simulink library "common_lib"  (R2021b)
settings: Solver=ode45  StartTime=0.0  StopTime=10.0  RelTol=1e-3
undefined symbols (not defined in the file or in its folder): ACCEL_PRE_MULT, C_C1GearNumbers, C_C1GearRatios, C_Calibration, C_DitherWaveform, C_GearOffset, C_GearRatioIn, C_GearRatioInverseOut, C_GearRatioOut, CLUTCH_INNER_LOOP_UPDATE_RATE, CONSTANT, DEGRADED_MODE_SIZE, Dem_EventStatusType, DiscIntNeverNeededParam, F_FAULT_ENUM, F_NOFAULT, F_OUTOFRANGE, F_RATELIMIT, FALSE, FMI14_SPECIAL_INSTRUCTIONS, FMI20_DATA_DRIFTED_HIGH, FMI21_DATA_DRIFTED_LOW, FMI29_RESERVED_FOR_SAE_ASSIGNMENT, FMI30_RESERVED_FOR_SAE_ASSIGNMENT, FMI31_CONDITION_EXISTS, FMI32_NO_FAULT, IC, k_accel, k_mean, LVDCU_OORH_FaultCntThd_C, MAX_UINT32, MEAN_PRE_MULT, NTriggers, QLTY_SIGNAL_FAILED, QLTY_SIGNAL_FULLY_FUNCTION, QLTY_SIGNAL_SUBSTITUTED_BY_1ST_CHOICE, QLTY_SIGNAL_SUBSTITUTED_BY_2ND_CHOICE, QLTY_SIGNAL_SUBSTITUTED_BY_3RD_CHOICE, QLTY_SIGNAL_SUBSTITUTED_BY_4TH_CHOICE, SAMPLE_TIME_100_mSec, SAMPLE_TIME_100_uSec, simin, T_TestPoint, TF_FALSE, TF_TRUE, TimeStep, TRUE, WORKSPACE_UPDATE_RATE, ZERO, Zero
libraries: $bdroot x120, simulink x27, simulink_extras x4, MBD_EPS_Local_Blockset x4
(part 4 of 10)

== system common_lib/Ctrl/Dither w Reset ==
  note: Filter output waveform to smooth
      | the transitions if necessary.
  note: Keep present output state until
      | number of executions has occured.
      | (initialize to FALSE)
  note: Keep track of number of iterations
      | since last output transition.
      | (initialize to zero)
  note: Calculate number of executions
      | between alternating output.
      | 1/ (2 * TimeStep * frequency)
      | Add in half a frame to roundoff to
      | nearest minor frame boundary
  note: Simple Dither Function
      | Outputs a modified rectangular wave of specified
      | amplitude, frequency and filter constant.  Also
      | provides a reset signal on switch of output sign.
  note: Common Library::Dither with Reset
  amplitude : Inport
  frequency : Inport  Port=2
  tau : Inport  Port=3
  Constant1 : Constant  Value=MinusOne
  Constant14 : Constant  Value=int16(1)
  Constant2 : Constant  Value=One
  Constant3 : Constant  Value=Two
  Constant4 : Constant  Value=One
  Constant5 : Constant  Value=lim
  Constant6 : Constant  Value=One
  Constant7 : Constant  Value=int16(1)
  Constant8 : Constant  Value=TimeStep
  Constant9 : Constant  Value=ZeroFive
  Data Type Conversion : DataTypeConversion  OutDataTypeStr=single  RndMeth=Zero
  Data Type Conversion1 : DataTypeConversion  OutDataTypeStr=single
  Fltr : $bdroot/Fltrs/Fltr  TimeStep=TimeStep
  Logical Operator : Logic  Operator=NOT
  Logical Operator1 : Logic  Operator=NOT
  MinMax1 : MinMax  Inputs=2  InputSameDT=on  SaturateOnIntegerOverflow=on  ZeroCross=off
  MinMax2 : MinMax  Function=max  Inputs=2  InputSameDT=on  SaturateOnIntegerOverflow=on  ZeroCross=off
  Product1 : Product  Inputs=**  InputSameDT=on  OutDataTypeStr=Inherit: Same as first input
  Product2 : Product  Inputs=***  InputSameDT=on  OutDataTypeStr=Inherit: Same as first input
  Product3 : Product  Inputs=*/  InputSameDT=on  OutDataTypeStr=Inherit: Same as first input
  Relational Operator : RelationalOperator  Operator=<  ZeroCross=off  RndMeth=Nearest  InputSameDT=on
  Sum1 : Sum  Inputs=|++  InputSameDT=on  OutDataTypeStr=Inherit: Same as first input
  Sum3 : Sum  Inputs=++|  InputSameDT=on  OutDataTypeStr=Inherit: Same as first input
  Switch1 : Switch  Threshold=0.5  ZeroCross=off  InputSameDT=on
  Switch2 : Switch  Threshold=0.5  ZeroCross=off  InputSameDT=on
  Switch3 : Switch  Threshold=0.5  ZeroCross=off  InputSameDT=on
  Unit Delay1 : UnitDelay  InitialCondition=int16(0)  SampleTime=-1  HasFrameUpgradeWarning=on
  Unit Delay11 : UnitDelay  InitialCondition=false  SampleTime=-1  HasFrameUpgradeWarning=on
  output : Outport  VectorParamsAs1DForOutWhenUnconnected=off
  reset : Outport  Port=2  VectorParamsAs1DForOutWhenUnconnected=off
  wires:
  Constant8/1 -> Data Type Conversion1/1
  Data Type Conversion1/1 -> Product2/1
  Constant9/1 -> Sum1/2
  Sum1/1 -> Relational Operator/2
  Data Type Conversion/1 -> Relational Operator/1
  Relational Operator/1 -> Logical Operator1/1, Switch1/2, Switch3/2
  Product3/1 -> Sum1/1
  Logical Operator/1 -> Switch1/3
  Sum3/1 -> Data Type Conversion/1, Switch3/1
  Constant7/1 -> Sum3/1
  Unit Delay1/1 -> Sum3/2
  Constant14/1 -> Switch3/3
  Switch3/1 -> Unit Delay1/1
  Constant3/1 -> Product2/3
  Constant6/1 -> Product3/1
  MinMax2/1 -> Product3/2
  Fltr/1 -> output/1
  Constant5/1 -> MinMax2/2
  MinMax1/1 -> MinMax2/1
  Constant4/1 -> MinMax1/2
  Product2/1 -> MinMax1/1
  frequency/1 -> Product2/2
  amplitude/1 -> Product1/1
  Switch2/1 -> Product1/2
  Constant2/1 -> Switch2/1
  Constant1/1 -> Switch2/3
  Product1/1 -> Fltr/1
  Switch1/1 -> Switch2/2, Unit Delay11/1
  Unit Delay11/1 -> Switch1/1, Logical Operator/1
  tau/1 -> Fltr/2
  Logical Operator1/1 -> reset/1

== system common_lib/Ctrl/Integrator ==
  note: Common Library::Integral
  input : Inport
  ulim : Inport  Port=2
  llim : Inport  Port=3
  ic : Inport  Port=4
  reset? : Inport  Port=5  OutDataTypeStr=boolean
  Constant1 : Constant  Value=TimeStep
  Data Type Conversion : DataTypeConversion  OutDataTypeStr=single
  Product1 : Product  Inputs=**  InputSameDT=on  OutDataTypeStr=Inherit: Same as first input
  Sat : $bdroot/Slink/Sat
  Sum : Sum  Inputs=++|  InputSameDT=on  OutDataTypeStr=Inherit: Same as first input
  Switch : Switch  Threshold=0.5  ZeroCross=off  InputSameDT=on
  Unit Delay : UnitDelay  InitialCondition=IC  SampleTime=-1  HasFrameUpgradeWarning=on
  Output : Outport  VectorParamsAs1DForOutWhenUnconnected=off
  wires:
  Constant1/1 -> Data Type Conversion/1
  Data Type Conversion/1 -> Product1/1
  Sat/1 -> Unit Delay/1, Output/1
  Unit Delay/1 -> Sum/1
  Switch/1 -> Sat/1
  Sum/1 -> Switch/3
  llim/1 -> Sat/3
  ulim/1 -> Sat/2
  reset?/1 -> Switch/2
  Product1/1 -> Sum/2
  ic/1 -> Switch/1
  input/1 -> Product1/2

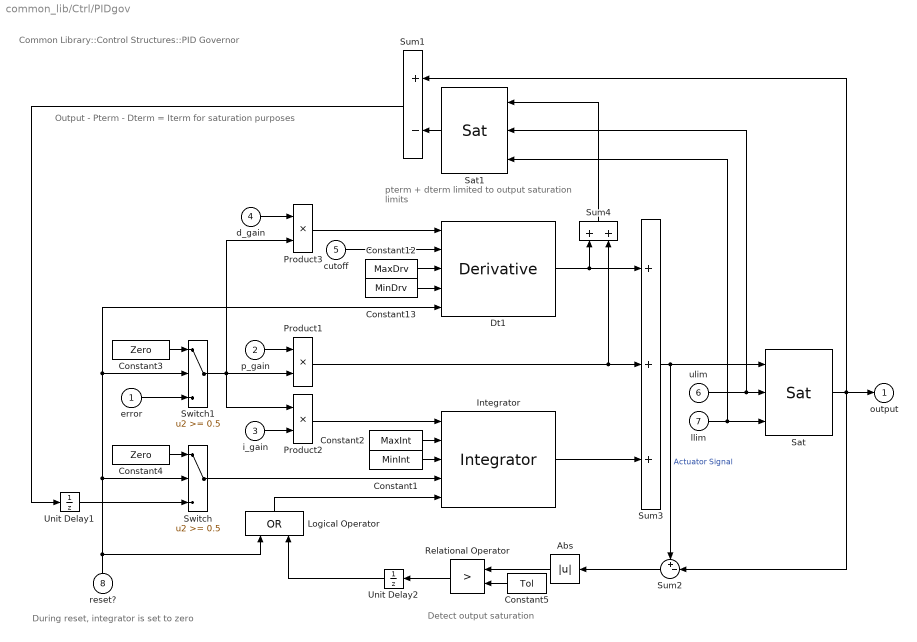
== system common_lib/Ctrl/PIDgov ==
  note: pterm + dterm
      | limited to output saturation limits
  note: Common Library::Control Structures::PID Governor
  note: Detect output saturation
  note: Output - Pterm - Dterm = Iterm for saturation purposes
  note: During reset, integrator is set to zero
  error : Inport
  p_gain : Inport  Port=2
  i_gain : Inport  Port=3
  d_gain : Inport  Port=4
  cutoff : Inport  Port=5
  ulim : Inport  Port=6
  llim : Inport  Port=7
  reset? : Inport  Port=8  OutDataTypeStr=boolean
  Abs : Abs  ZeroCross=off
  Constant1 : Constant  Value=MinInt
  Constant12 : Constant  Value=MaxDrv
  Constant13 : Constant  Value=MinDrv
  Constant2 : Constant  Value=MaxInt
  Constant3 : Constant  Value=Zero
  Constant4 : Constant  Value=Zero
  Constant5 : Constant  Value=Tol
  Dt1 : $bdroot/Ctrl/Derivative  TimeStep=TimeStep
  Integrator : $bdroot/Ctrl/Integrator  TimeStep=TimeStep  IC=IC
  Logical Operator : Logic  Operator=OR
  Product1 : Product  InputSameDT=on  OutDataTypeStr=Inherit: Same as first input
  Product2 : Product  InputSameDT=on  OutDataTypeStr=Inherit: Same as first input
  Product3 : Product  InputSameDT=on  OutDataTypeStr=Inherit: Same as first input
  Relational Operator : RelationalOperator  Operator=>  ZeroCross=off  RndMeth=Nearest  InputSameDT=on
  Sat : $bdroot/Slink/Sat
  Sat1 : $bdroot/Slink/Sat
  Sum1 : Sum  Inputs=+-  InputSameDT=on  OutDataTypeStr=Inherit: Same as first input
  Sum2 : Sum  Inputs=+-|  InputSameDT=on  OutDataTypeStr=Inherit: Same as first input
  Sum3 : Sum  Inputs=+++  InputSameDT=on  OutDataTypeStr=Inherit: Same as first input
  Sum4 : Sum  InputSameDT=on  OutDataTypeStr=Inherit: Same as first input
  Switch : Switch  Threshold=0.5  ZeroCross=off  InputSameDT=on
  Switch1 : Switch  Threshold=0.5  ZeroCross=off  InputSameDT=on
  Unit Delay1 : UnitDelay  InitialCondition=Zero  SampleTime=-1  HasFrameUpgradeWarning=on
      settings: AttributesFormatString=ic=%<X0>
  Unit Delay2 : UnitDelay  InitialCondition=false  SampleTime=-1  HasFrameUpgradeWarning=on
      settings: AttributesFormatString=ic=%<X0>
  output : Outport  InitialOutput=8.973  VectorParamsAs1DForOutWhenUnconnected=off
  wires:
  Switch1/1 -> Product1/2, Product2/1, Product3/2
  error/1 -> Switch1/3
  Constant3/1 -> Switch1/1
  cutoff/1 -> Dt1/2
  Constant12/1 -> Dt1/3
  Constant13/1 -> Dt1/4
  Sat1/1 -> Sum1/2
  Sum4/1 -> Sat1/1
  Dt1/1 -> Sum3/1, Sum4/1
  Unit Delay1/1 -> Switch/3
  Sum2/1 -> Abs/1
  Relational Operator/1 -> Unit Delay2/1
  Abs/1 -> Relational Operator/1
  Constant5/1 -> Relational Operator/2
  Constant2/1 -> Integrator/2
  Constant1/1 -> Integrator/3
  reset?/1 -> Switch1/2, Dt1/5, Switch/2, Logical Operator/1
  ulim/1 -> Sat1/2, Sat/2
  p_gain/1 -> Product1/1
  Product1/1 -> Sum3/2, Sum4/2
  llim/1 -> Sat1/3, Sat/3
  Sum3/1 -> Sat/1, Sum2/1  "Actuator Signal"
  Sat/1 -> Sum1/1, output/1, Sum2/2
  i_gain/1 -> Product2/2
  Constant4/1 -> Switch/1
  Logical Operator/1 -> Integrator/5
  Unit Delay2/1 -> Logical Operator/2
  Switch/1 -> Integrator/4
  Integrator/1 -> Sum3/3
  Sum1/1 -> Unit Delay1/1
  Product2/1 -> Integrator/1
  Product3/1 -> Dt1/1
  d_gain/1 -> Product3/1

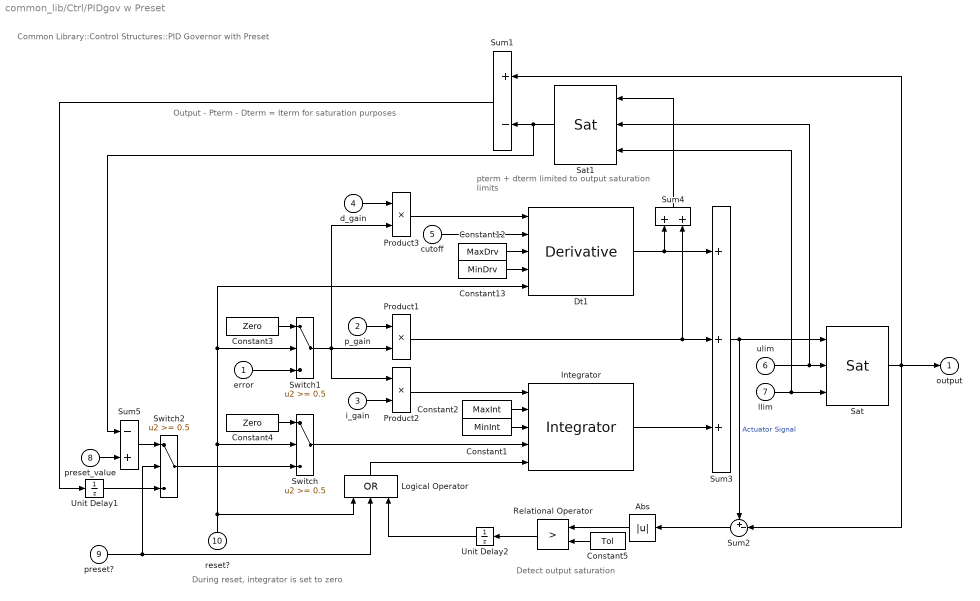
== system common_lib/Ctrl/PIDgov w Preset ==
  note: pterm + dterm
      | limited to output saturation limits
  note: Common Library::Control Structures::PID Governor with Preset
  note: Detect output saturation
  note: Output - Pterm - Dterm = Iterm for saturation purposes
  note: During reset, integrator is set to zero
  error : Inport
  p_gain : Inport  Port=2
  i_gain : Inport  Port=3
  d_gain : Inport  Port=4
  cutoff : Inport  Port=5
  ulim : Inport  Port=6
  llim : Inport  Port=7
  preset_value : Inport  Port=8
  preset? : Inport  Port=9
  reset? : Inport  Port=10  OutDataTypeStr=boolean
  Abs : Abs  ZeroCross=off
  Constant1 : Constant  Value=MinInt
  Constant12 : Constant  Value=MaxDrv
  Constant13 : Constant  Value=MinDrv
  Constant2 : Constant  Value=MaxInt
  Constant3 : Constant  Value=Zero
  Constant4 : Constant  Value=Zero
  Constant5 : Constant  Value=Tol
  Dt1 : $bdroot/Ctrl/Derivative  TimeStep=TimeStep
  Integrator : $bdroot/Ctrl/Integrator  TimeStep=TimeStep  IC=IC
  Logical Operator : Logic  Operator=OR  Inputs=3
  Product1 : Product  InputSameDT=on  OutDataTypeStr=Inherit: Same as first input
  Product2 : Product  InputSameDT=on  OutDataTypeStr=Inherit: Same as first input
  Product3 : Product  InputSameDT=on  OutDataTypeStr=Inherit: Same as first input
  Relational Operator : RelationalOperator  Operator=>  ZeroCross=off  RndMeth=Nearest  InputSameDT=on
  Sat : $bdroot/Slink/Sat
  Sat1 : $bdroot/Slink/Sat
  Sum1 : Sum  Inputs=+-  InputSameDT=on  OutDataTypeStr=Inherit: Same as first input
  Sum2 : Sum  Inputs=+-|  InputSameDT=on  OutDataTypeStr=Inherit: Same as first input
  Sum3 : Sum  Inputs=+++  InputSameDT=on  OutDataTypeStr=Inherit: Same as first input
  Sum4 : Sum  InputSameDT=on  OutDataTypeStr=Inherit: Same as first input
  Sum5 : Sum  Inputs=-+  InputSameDT=on  OutDataTypeStr=Inherit: Same as first input
  Switch : Switch  Threshold=0.5  ZeroCross=off  InputSameDT=on
  Switch1 : Switch  Threshold=0.5  ZeroCross=off  InputSameDT=on
  Switch2 : Switch  Threshold=0.5  ZeroCross=off  InputSameDT=on
  Unit Delay1 : UnitDelay  InitialCondition=Zero  SampleTime=-1  HasFrameUpgradeWarning=on
      settings: AttributesFormatString=ic=%<X0>
  Unit Delay2 : UnitDelay  InitialCondition=false  SampleTime=-1  HasFrameUpgradeWarning=on
      settings: AttributesFormatString=ic=%<X0>
  output : Outport  InitialOutput=8.973  VectorParamsAs1DForOutWhenUnconnected=off
  wires:
  Sum5/1 -> Switch2/1
  preset_value/1 -> Sum5/2
  Switch2/1 -> Switch/3
  Unit Delay1/1 -> Switch2/3
  Switch1/1 -> Product1/2, Product2/1, Product3/2
  error/1 -> Switch1/3
  Constant3/1 -> Switch1/1
  cutoff/1 -> Dt1/2
  Constant12/1 -> Dt1/3
  Constant13/1 -> Dt1/4
  preset?/1 -> Switch2/2, Logical Operator/2
  Sat1/1 -> Sum5/1, Sum1/2
  Sum4/1 -> Sat1/1
  Dt1/1 -> Sum3/1, Sum4/1
  Sum2/1 -> Abs/1
  Relational Operator/1 -> Unit Delay2/1
  Abs/1 -> Relational Operator/1
  Constant5/1 -> Relational Operator/2
  Constant2/1 -> Integrator/2
  Constant1/1 -> Integrator/3
  reset?/1 -> Switch1/2, Dt1/5, Switch/2, Logical Operator/1
  ulim/1 -> Sat1/2, Sat/2
  p_gain/1 -> Product1/1
  Product1/1 -> Sum3/2, Sum4/2
  llim/1 -> Sat1/3, Sat/3
  Sum3/1 -> Sat/1, Sum2/1  "Actuator Signal"
  Sat/1 -> Sum1/1, output/1, Sum2/2
  i_gain/1 -> Product2/2
  Constant4/1 -> Switch/1
  Logical Operator/1 -> Integrator/5
  Unit Delay2/1 -> Logical Operator/3
  Switch/1 -> Integrator/4
  Integrator/1 -> Sum3/3
  Sum1/1 -> Unit Delay1/1
  Product2/1 -> Integrator/1
  Product3/1 -> Dt1/1
  d_gain/1 -> Product3/1

== system common_lib/Ctrl/PIgov ==
  note: pterm
      | limited to output saturation limits
  note: Common Library::Control Structures::PI Governor
  note: Detect output saturation
  note: Output - Pterm - Dterm = Iterm for saturation purposes
  note: During reset, integrator is set to zero
  error : Inport
  p_gain : Inport  Port=2
  i_gain : Inport  Port=3
  ulim : Inport  Port=4
  llim : Inport  Port=5
  reset? : Inport  Port=6  OutDataTypeStr=boolean
  Abs : Abs  ZeroCross=off
  Constant1 : Constant  Value=MinInt
  Constant2 : Constant  Value=MaxInt
  Constant3 : Constant  Value=Zero  OutDataTypeStr=Inherit: Inherit via back propagation
  Constant4 : Constant  Value=Zero  OutDataTypeStr=Inherit: Inherit via back propagation
  Constant5 : Constant  Value=Tol
  Integrator01 : Subsystem  AncestorBlock=common_lib/Ctrl/Integrator  TreatAsAtomicUnit=on  RTWFcnName=INTEGRATOR01  mask(CL Integrator){TimeStep=TimeStep, IC=IC}
      mask prompts: TimeStep "Time Step"; IC "Initial Condition"
      mask help:
      | Determine the integral of the input.
      | If reset is true (1), the integrator is set to the reset condition input.
      |
      | X(1) = input
      | X(2) = upper limit
      | X(3) = lower limit
      | X(4) = reset condition
      | X(5) = reset
      |
      | Y(1) = output
      |
      | Time step is entered via mask parameter.
      | Initial condition is entered via mask parameter.
      |
      | NgEK, Inc.
      settings: RTWFcnNameOpts=User specified  RTWFileNameOpts=Use function name
      mask Help: web(which(['common_lib3.html']))
      mask Display:
      | patch([0.3 0.3 0.7 0.7], [0.35 0.65 0.65 0.35], [255/255 127/255 255/255])
      | disp('Integrator')
      | port_label('input', 1, 'input')
      | port_label('input', 2, 'ulim')
      | port_label('input', 3, 'llim')
      | port_label('input', 4, 'reset_cond')
      | port_label('input', 5, 'reset?')
      | port_label('output', 1, 'output')
  Logical Operator : Logic  Operator=OR
  Product1 : Product  InputSameDT=on  OutDataTypeStr=Inherit: Same as first input
  Product2 : Product  InputSameDT=on  OutDataTypeStr=Inherit: Same as first input
  Relational Operator : RelationalOperator  Operator=>  ZeroCross=off  RndMeth=Nearest  InputSameDT=on
  Sat : $bdroot/Slink/Sat
  Sat1 : $bdroot/Slink/Sat
  Sum1 : Sum  Inputs=+-  InputSameDT=on  OutDataTypeStr=Inherit: Same as first input
  Sum2 : Sum  Inputs=+-|  InputSameDT=on  OutDataTypeStr=Inherit: Same as first input
  Sum3 : Sum  InputSameDT=on  OutDataTypeStr=Inherit: Same as first input
  Switch : Switch  Threshold=0.5  ZeroCross=off  InputSameDT=on
  Switch1 : Switch  Threshold=0.5  ZeroCross=off  InputSameDT=on
  Unit Delay1 : UnitDelay  InitialCondition=Zero  SampleTime=-1  HasFrameUpgradeWarning=on
      settings: AttributesFormatString=ic=%<X0>
  Unit Delay2 : UnitDelay  InitialCondition=false  SampleTime=-1  HasFrameUpgradeWarning=on
      settings: AttributesFormatString=ic=%<X0>
  output : Outport  InitialOutput=8.973  VectorParamsAs1DForOutWhenUnconnected=off
  wires:
  Switch1/1 -> Product1/2, Product2/1
  error/1 -> Switch1/3
  Constant3/1 -> Switch1/1
  Sat1/1 -> Sum1/2
  Unit Delay1/1 -> Switch/3
  Sum2/1 -> Abs/1
  Relational Operator/1 -> Unit Delay2/1
  Abs/1 -> Relational Operator/1
  Constant5/1 -> Relational Operator/2
  Constant2/1 -> Integrator01/2(ulim)
  Constant1/1 -> Integrator01/3(llim)
  reset?/1 -> Logical Operator/1, Switch1/2, Switch/2
  ulim/1 -> Sat1/2, Sat/2
  p_gain/1 -> Product1/1
  Product1/1 -> Sum3/1, Sat1/1
  llim/1 -> Sat1/3, Sat/3
  Sum3/1 -> Sat/1, Sum2/1  "Actuator Signal"
  Sat/1 -> Sum1/1, output/1, Sum2/2
  i_gain/1 -> Product2/2
  Constant4/1 -> Switch/1
  Logical Operator/1 -> Integrator01/5(reset?)
  Unit Delay2/1 -> Logical Operator/2
  Switch/1 -> Integrator01/4(ic)
  Integrator01/1(Output) -> Sum3/2
  Sum1/1 -> Unit Delay1/1
  Product2/1 -> Integrator01/1(input)

== system common_lib/Ctrl/PIgov w Preset ==
  note: pterm
      | limited to output saturation limits
  note: Common Library::Control Structures::PID Governor with Preset
  note: Detect output saturation
  note: Output - Pterm - Dterm = Iterm for saturation purposes
  note: During reset, integrator is set to zero
  error : Inport
  p_gain : Inport  Port=2
  i_gain : Inport  Port=3
  ulim : Inport  Port=4
  llim : Inport  Port=5
  preset_value : Inport  Port=6
  preset? : Inport  Port=7
  reset? : Inport  Port=8  OutDataTypeStr=boolean
  Abs : Abs  ZeroCross=off
  Constant1 : Constant  Value=MinInt
  Constant2 : Constant  Value=MaxInt
  Constant3 : Constant  Value=Zero
  Constant4 : Constant  Value=Zero
  Constant5 : Constant  Value=Tol
  Integrator : $bdroot/Ctrl/Integrator  TimeStep=TimeStep  IC=IC
  Logical Operator : Logic  Operator=OR  Inputs=3
  Product1 : Product  InputSameDT=on  OutDataTypeStr=Inherit: Same as first input
  Product2 : Product  InputSameDT=on  OutDataTypeStr=Inherit: Same as first input
  Relational Operator : RelationalOperator  Operator=>  ZeroCross=off  RndMeth=Nearest  InputSameDT=on
  Sat : $bdroot/Slink/Sat
  Sat1 : $bdroot/Slink/Sat
  Sum1 : Sum  Inputs=+-  InputSameDT=on  OutDataTypeStr=Inherit: Same as first input
  Sum2 : Sum  Inputs=+-|  InputSameDT=on  OutDataTypeStr=Inherit: Same as first input
  Sum3 : Sum  InputSameDT=on  OutDataTypeStr=Inherit: Same as first input
  Sum4 : Sum  Inputs=-+  InputSameDT=on  OutDataTypeStr=Inherit: Same as first input
  Switch : Switch  Threshold=0.5  ZeroCross=off  InputSameDT=on
  Switch1 : Switch  Threshold=0.5  ZeroCross=off  InputSameDT=on
  Switch2 : Switch  Threshold=0.5  ZeroCross=off  InputSameDT=on
  Unit Delay1 : UnitDelay  InitialCondition=Zero  SampleTime=-1  HasFrameUpgradeWarning=on
      settings: AttributesFormatString=ic=%<X0>
  Unit Delay2 : UnitDelay  InitialCondition=false  SampleTime=-1  HasFrameUpgradeWarning=on
      settings: AttributesFormatString=ic=%<X0>
  output : Outport  InitialOutput=8.973  VectorParamsAs1DForOutWhenUnconnected=off
  wires:
  Sum4/1 -> Switch2/1
  Switch2/1 -> Switch/3
  preset_value/1 -> Sum4/2
  Unit Delay1/1 -> Switch2/3
  Switch1/1 -> Product1/2, Product2/1
  error/1 -> Switch1/3
  Constant3/1 -> Switch1/1
  preset?/1 -> Switch2/2, Logical Operator/2
  Sat1/1 -> Sum4/1, Sum1/2
  Sum2/1 -> Abs/1
  Relational Operator/1 -> Unit Delay2/1
  Abs/1 -> Relational Operator/1
  Constant5/1 -> Relational Operator/2
  Constant2/1 -> Integrator/2
  Constant1/1 -> Integrator/3
  reset?/1 -> Switch1/2, Switch/2, Logical Operator/1
  ulim/1 -> Sat1/2, Sat/2
  p_gain/1 -> Product1/1
  Product1/1 -> Sum3/1, Sat1/1
  llim/1 -> Sat1/3, Sat/3
  Sum3/1 -> Sat/1, Sum2/1  "Actuator Signal"
  Sat/1 -> Sum1/1, output/1, Sum2/2
  i_gain/1 -> Product2/2
  Constant4/1 -> Switch/1
  Logical Operator/1 -> Integrator/5
  Unit Delay2/1 -> Logical Operator/3
  Switch/1 -> Integrator/4
  Integrator/1 -> Sum3/2
  Sum1/1 -> Unit Delay1/1
  Product2/1 -> Integrator/1

== system common_lib/Ctrl/Ramp ==
  note: Common Library::Ramp
  A : Inport
  B : Inport  Port=2
  C : Inport  Port=3
  reset : Inport  Port=4  OutDataTypeStr=boolean
  Constant1 : Constant  Value=TimeStep
  Data Type Conversion : DataTypeConversion  OutDataTypeStr=single
  MinMax1 : MinMax  Function=max  Inputs=2  InputSameDT=on  SaturateOnIntegerOverflow=on  ZeroCross=off
  MinMax2 : MinMax  Function=max  Inputs=2  InputSameDT=on  SaturateOnIntegerOverflow=on  ZeroCross=off
  MinMax3 : MinMax  Inputs=2  InputSameDT=on  SaturateOnIntegerOverflow=on  ZeroCross=off
  Product1 : Product  Inputs=/**  InputSameDT=on  OutDataTypeStr=Inherit: Same as first input
  Sat : $bdroot/Slink/Sat
  Sum : Sum  Inputs=++|  InputSameDT=on  OutDataTypeStr=Inherit: Same as first input
  Sum1 : Sum  Inputs=-|+  InputSameDT=on  OutDataTypeStr=Inherit: Same as first input
  Switch : Switch  Threshold=0.5  ZeroCross=off  InputSameDT=on
  Switch1 : Switch  Threshold=0.5  ZeroCross=off  InputSameDT=on
  Unit Delay : UnitDelay  InitialCondition=Zero  SampleTime=-1  HasFrameUpgradeWarning=on
      settings: AttributesFormatString=ic=%<X0>
  Unit Delay1 : UnitDelay  InitialCondition=Zero  SampleTime=-1  HasFrameUpgradeWarning=on
      settings: AttributesFormatString=ic=%<X0>
  Unit Delay2 : UnitDelay  InitialCondition=true  SampleTime=-1  HasFrameUpgradeWarning=on
      settings: AttributesFormatString=ic=%<X0>
  Output : Outport  VectorParamsAs1DForOutWhenUnconnected=off
  wires:
  Data Type Conversion/1 -> MinMax1/2, Product1/2
  Constant1/1 -> Data Type Conversion/1
  Unit Delay2/1 -> Switch1/2
  reset/1 -> Unit Delay2/1, Switch/2
  Product1/1 -> Sum/2
  Switch1/1 -> Product1/3, Unit Delay1/1
  Sum1/1 -> Switch1/1
  Unit Delay1/1 -> Switch1/3
  MinMax3/1 -> Sat/3
  MinMax2/1 -> Sat/2
  MinMax1/1 -> Product1/1
  C/1 -> MinMax1/1
  Sat/1 -> Unit Delay/1, Output/1
  Unit Delay/1 -> Sum/1
  Switch/1 -> Sat/1
  Sum/1 -> Switch/3
  B/1 -> MinMax2/2, MinMax3/2, Sum1/2
  A/1 -> MinMax3/1, MinMax2/1, Sum1/1, Switch/1

== system common_lib/Ctrl/Subsystem ==
  ClearCntrRqst : Inport
  Increment_Cntr : Inport  Port=2
  HWpd_Input : Inport  Port=3
  Constant15 : Constant  Value=uint32(1)
  Constant16 : Constant  Value=FALSE
  Constant17 : Constant  Value=MAX_UINT32
  Constant18 : Constant  Value=uint32(0)
  Constant19 : Constant  Value=uint32(0)
  Logical Operator9 : Logic  AllPortsSameDT=off
  Relational Operator6 : RelationalOperator  Operator=<  ZeroCross=off  RndMeth=Nearest  InputSameDT=on
  Sum4 : Sum  Inputs=|++  InputSameDT=on  OutDataTypeStr=Inherit: Same as first input
  Switch10 : Switch  Threshold=0.5  ZeroCross=off  InputSameDT=on
  Switch11 : Switch  Threshold=0.5  ZeroCross=off  InputSameDT=on
  Switch12 : Switch  Threshold=0.5  ZeroCross=off  InputSameDT=on
  Unit Delay8 : UnitDelay  InitialCondition=uint32(0)  SampleTime=-1  HasFrameUpgradeWarning=on
      settings: AttributesFormatString=ic=%<X0>
  Unit Delay9 : UnitDelay  InitialCondition=TRUE  SampleTime=-1  HasFrameUpgradeWarning=on
      settings: AttributesFormatString=ic=%<X0>
  CntrUpdate : Outport  VectorParamsAs1DForOutWhenUnconnected=off
  wires:
  Unit Delay8/1 -> Relational Operator6/1, Sum4/2
  Constant17/1 -> Relational Operator6/2
  Constant19/1 -> Switch12/1
  Switch10/1 -> Switch12/3
  Constant18/1 -> Switch11/3
  Constant15/1 -> Switch11/1
  Switch11/1 -> Sum4/1
  Sum4/1 -> Switch10/3
  Unit Delay9/1 -> Switch10/2
  Constant16/1 -> Unit Delay9/1
  Switch12/1 -> Unit Delay8/1, CntrUpdate/1
  Logical Operator9/1 -> Switch11/2
  Increment_Cntr/1 -> Logical Operator9/1
  Relational Operator6/1 -> Logical Operator9/2
  HWpd_Input/1 -> Switch10/1
  ClearCntrRqst/1 -> Switch12/2

== system common_lib/Ctrl/Trajectory ==
  note: Rate increment happens
      | even during reset
  note: Output - Final
  note: Start - Final
  note: Ignore the start_value
      | if it is moving away
      | from the final_value
  note: Reset if the previous value is further
      |                       away than the current start value
      | or if the final limit is smaller than the start limit
      | or if start is active
  note: Pick rate based on distance
      | from final
  note: Pick rate based on distance
      | from original start
  note: Start-CurrentStart
  note: Common Library::Control Structures::Trajectory Control
  start_value : Inport
  final_value : Inport  Port=2
  start_weight : Inport  Port=3
  stop_weight : Inport  Port=4
  start : Inport  Port=5
  Abs{,1,3..5} (5 alike) : Abs  ZeroCross=off
  Constant1 : Constant  Value=MinusOne
  CurrentStart : Subsystem  TreatAsAtomicUnit=on
      settings: RTWSystemCode=Inline
  FinalRLim : Lookup  InputValues=FinalRLimIn  Table=FinalRLimOut  LookUpMeth=Interpolation-Use End Values
  Logical Operator : Logic  Operator=OR  Inputs=3
  Logical Operator1 : Logic  Operator=OR
  MinMax3 : MinMax  Inputs=2  InputSameDT=on  SaturateOnIntegerOverflow=on  ZeroCross=off
  Relational Operator : RelationalOperator  Operator=<  ZeroCross=off  RndMeth=Nearest  InputSameDT=on
  Relational Operator1 : RelationalOperator  Operator=>  ZeroCross=off  RndMeth=Nearest  InputSameDT=on
  Relational Operator2 : RelationalOperator  ZeroCross=off  RndMeth=Nearest  InputSameDT=on
  Start : Subsystem  TreatAsAtomicUnit=on
      settings: RTWSystemCode=Inline
  StartRLim : Lookup  InputValues=StartRLimIn  Table=StartRLimOut  LookUpMeth=Interpolation-Use End Values
  Sum1 : Sum  Inputs=-+  InputSameDT=on  OutDataTypeStr=Inherit: Same as first input
  Sum2 : Sum  Inputs=-+  InputSameDT=on  OutDataTypeStr=Inherit: Same as first input
  Sum3 : Sum  Inputs=+-  InputSameDT=on  OutDataTypeStr=Inherit: Same as first input
  Sum4 : Sum  Inputs=+-  InputSameDT=on  OutDataTypeStr=Inherit: Same as first input
  Sum6 : Sum  Inputs=+-  InputSameDT=on  OutDataTypeStr=Inherit: Same as first input
  Unit Delay1 : UnitDelay  InitialCondition=Zero  SampleTime=-1  HasFrameUpgradeWarning=on
      settings: AttributesFormatString=ic=%<X0>
  Unit Delay2 : UnitDelay  InitialCondition=Zero  SampleTime=-1  HasFrameUpgradeWarning=on
      settings: AttributesFormatString=ic=%<X0>
  Variable Rate Limiter w IC in feedback loop : Subsystem  mask(CL Variable Rate Limiter with Initial Condition){TimeStep=TimeStep, ic=Zero}
      mask prompts: TimeStep "Time Step"; ic "Initial Condition"
      mask help:
      | Variable rate limiter block with Initial Condiiton
      |
      | X(1) = input
      | X(2) = rise rate
      | X(3) = fall rate
      | X(4) = initial condition
      | X(5) = reset?
      |
      | Y(1) = output
      | NgEK, Inc.
      mask Help: web(which(['common_lib38.html']))
      mask Display:
      | patch([0.3 0.3 0.7 0.7], [0.35 0.65 0.65 0.35], [255/255 127/255 255/255])
      | 
      | plot([0 1],[0.5 0.5],[0.5 0.5],[0 1],[0 1],[0 1],[0.7 0.8 0.8],[0.8 0.8 0.7], [0.2 0.2 0.3],[0.3 0.2 0.2])
  transient_split3 : Product  InputSameDT=on  OutDataTypeStr=Inherit: Same as first input
  transient_split5 : Product  InputSameDT=on  OutDataTypeStr=Inherit: Same as first input
  transient_split6 : Product  InputSameDT=on  OutDataTypeStr=Inherit: Same as first input
  output : Outport  VectorParamsAs1DForOutWhenUnconnected=off
  wires:
  Abs5/1 -> Relational Operator2/1
  Sum4/1 -> Abs5/1
  Unit Delay2/1 -> Sum4/1
  Abs4/1 -> Relational Operator2/2
  Sum3/1 -> Abs4/1
  Relational Operator2/1 -> Logical Operator1/1
  Logical Operator1/1 -> CurrentStart/Enable
  CurrentStart/1(out) -> Start/1(in), Sum1/1, Unit Delay2/1, Variable Rate Limiter w IC in feedback loop/4(ic), Sum2/2
  Variable Rate Limiter w IC in feedback loop/1(output) -> Unit Delay1/1, output/1
  Relational Operator1/1 -> Logical Operator/1
  Abs3/1 -> Relational Operator1/1
  Sum6/1 -> Abs3/1
  Logical Operator/1 -> Variable Rate Limiter w IC in feedback loop/5(reset?)
  Unit Delay1/1 -> Sum6/1
  Relational Operator/1 -> Logical Operator/2
  transient_split5/1 -> Variable Rate Limiter w IC in feedback loop/3(fall rate)
  MinMax3/1 -> Variable Rate Limiter w IC in feedback loop/2(rise rate), transient_split5/1
  final_value/1 -> Sum4/2, Sum3/1, Variable Rate Limiter w IC in feedback loop/1(input), Sum6/2, Sum2/1
  transient_split6/1 -> Relational Operator/1, MinMax3/1
  FinalRLim/1 -> transient_split6/2
  Abs1/1 -> Relational Operator1/2, FinalRLim/1
  Sum2/1 -> Abs1/1
  Constant1/1 -> transient_split5/2
  stop_weight/1 -> transient_split6/1
  transient_split3/1 -> Relational Operator/2, MinMax3/2
  StartRLim/1 -> transient_split3/2
  Abs/1 -> StartRLim/1
  Sum1/1 -> Abs/1
  Start/1(out) -> Sum1/2
  start_weight/1 -> transient_split3/1
  start/1 -> Start/Enable, Logical Operator/3, Logical Operator1/2
  start_value/1 -> CurrentStart/1(in), Sum3/2

== system common_lib/Ctrl/VoltageControllerPI ==
  Err : Inport  OutDataTypeStr=single
  reset : Inport  Port=2  OutDataTypeStr=boolean
  b0 : Inport  Port=3  OutDataTypeStr=single
  b1 : Inport  Port=4  OutDataTypeStr=single
  Add : Sum  Inputs=+++  SaturateOnIntegerOverflow=on
  Constant : Constant  Value=0  OutDataTypeStr=single  SampleTime=-1
  Constant1 : Constant  Value=0  OutDataTypeStr=single  SampleTime=-1
  Divide : Product
  Divide1 : Product
  Saturation : Saturate  UpperLimit=ul  LowerLimit=ll  OutDataTypeStr=single
  Switch : Switch  Criteria=u2 > Threshold  Threshold=0.5
  Switch1 : Switch  Criteria=u2 > Threshold  Threshold=0.5
  Unit Delay : UnitDelay  SampleTime=-1  HasFrameUpgradeWarning=on
      settings: AttributesFormatString=ic=%<X0>
  Unit Delay1 : UnitDelay  SampleTime=-1  HasFrameUpgradeWarning=on
      settings: AttributesFormatString=ic=%<X0>
  out : Outport  VectorParamsAs1DForOutWhenUnconnected=off
  wires:
  Unit Delay/1 -> Divide1/1
  Divide/1 -> Add/1
  Divide1/1 -> Add/2
  Add/1 -> Saturation/1
  Saturation/1 -> Unit Delay1/1, out/1
  Unit Delay1/1 -> Switch/3
  Switch/1 -> Add/3
  reset/1 -> [Reset]
  Constant/1 -> Switch/1
  [Reset] -> Switch/2
  Err/1 -> Switch1/3
  Switch1/1 -> Unit Delay/1, Divide/2
  [Reset] -> Switch1/2
  Constant1/1 -> Switch1/1
  b0/1 -> Divide/1
  b1/1 -> Divide1/2

== system common_lib/Diag/CL MinMax Capture ==
  input : Inport
  hold? : Inport  Port=2
  reset? : Inport  Port=3
  Constant : Constant  Value=InitValue  SampleTime=-1
  Logical Operator : Logic  AllPortsSameDT=off
  Logical Operator1 : Logic  Operator=NOT  AllPortsSameDT=off
  Relational Operator : RelationalOperator  Operator=<  ZeroCross=off  RndMeth=Nearest
  Switch : Switch  Threshold=0.5  ZeroCross=off
  Switch1 : Switch  Threshold=0.5  ZeroCross=off
  Unit Delay : UnitDelay  InitialCondition=InitValue  SampleTime=-1  HasFrameUpgradeWarning=on
      settings: AttributesFormatString=ic=%<X0>
  Output Value : Outport  VectorParamsAs1DForOutWhenUnconnected=off
  wires:
  Constant/1 -> Switch/1
  reset?/1 -> Switch/2
  Switch1/1 -> Switch/3
  input/1 -> Switch1/1, Relational Operator/1  "Input"
  Relational Operator/1 -> Logical Operator/2  "Input past previous value"
  hold?/1 -> Logical Operator1/1  "Hold value"
  Logical Operator1/1 -> Logical Operator/1
  Logical Operator/1 -> Switch1/2  "New value"
  Switch/1 -> Unit Delay/1, Output Value/1
  Unit Delay/1 -> Switch1/3, Relational Operator/2  "Previous value"

== system common_lib/Diag/Command Feedback Test ==
  note: Common Library::Diagnostics::Command Feedback Test
  cmd : Inport
  fbk : Inport  Port=2
  tau : Inport  Port=3
  tau_lim : Inport  Port=4
  tau_time : Inport  Port=5
  error_lim : Inport  Port=6
  error_time : Inport  Port=7
  Enable : EnablePort  ZeroCross=off
  CommandFeedbackFaultLogicCore : Subsystem  TreatAsAtomicUnit=on  RTWFcnName=CFT
      settings: RTWFcnNameOpts=User specified  RTWFileNameOpts=Use function name
  Data Type Conversion{1..7} (7 alike) : DataTypeConversion  OutDataTypeStr=single
  Signal Conversion : SignalConversion  ConversionOutput=Contiguous copy  OverrideOpt=on
  Min Value : Outport  VectorParamsAs1DForOutWhenUnconnected=off
  wires:
  cmd/1 -> Data Type Conversion7/1
  tau/1 -> Data Type Conversion5/1
  tau_lim/1 -> Data Type Conversion4/1
  tau_time/1 -> Data Type Conversion3/1
  error_lim/1 -> Data Type Conversion2/1
  CommandFeedbackFaultLogicCore/1(Min Value) -> Signal Conversion/1
  fbk/1 -> Data Type Conversion6/1
  error_time/1 -> Data Type Conversion1/1
  Signal Conversion/1 -> Min Value/1
  Data Type Conversion1/1 -> CommandFeedbackFaultLogicCore/7(error_time)
  Data Type Conversion2/1 -> CommandFeedbackFaultLogicCore/6(error_lim)
  Data Type Conversion3/1 -> CommandFeedbackFaultLogicCore/5(tau_time)
  Data Type Conversion4/1 -> CommandFeedbackFaultLogicCore/4(tau_lim)
  Data Type Conversion5/1 -> CommandFeedbackFaultLogicCore/3(tau)
  Data Type Conversion6/1 -> CommandFeedbackFaultLogicCore/2(fbk)
  Data Type Conversion7/1 -> CommandFeedbackFaultLogicCore/1(cmd)

== system common_lib/Diag/Fault Counter ==
  note: Common Library::Diagnostics::Fault Counter
  fl : Inport  OutDataTypeStr=boolean
  true_count : Inport  Port=2
  false_count : Inport  Port=3
  fc_level : Inport  Port=4
  reset : Inport  Port=5  OutDataTypeStr=boolean
  Compare To Zero : simulink/Logic and Bit Operations/Compare To Zero  relop=>  OutDataTypeStr=boolean  ZeroCross=off
  Constant : Constant  Value=true
  DTC : DataTypeConversion  OutDataTypeStr=boolean
  DTC1 : DataTypeConversion  OutDataTypeStr=boolean
  DTC3 : DataTypeConversion  OutDataTypeStr=int16
  FaultCounter : Subsystem  RTWFcnName=FLTCNTR
      settings: RTWSystemCode=Inline  RTWFcnNameOpts=User specified  RTWFileNameOpts=Use function name
  Logical Operator : Logic  AllPortsSameDT=off  OutDataTypeStr=boolean
  Logical Operator1 : Logic  Operator=OR  AllPortsSameDT=off  OutDataTypeStr=boolean
  Signal Conversion : SignalConversion  ConversionOutput=Contiguous copy  OverrideOpt=on
  Unit Delay : UnitDelay  InitialCondition=ZERO  SampleTime=-1  HasFrameUpgradeWarning=on
      settings: AttributesFormatString=ic=%<X0>
  Unit Delay1 : UnitDelay  InitialCondition=false  SampleTime=-1  HasFrameUpgradeWarning=on
      settings: AttributesFormatString=ic=%<X0>
  inc switch : Switch  Criteria=u2 ~= 0  Threshold=0.5  ZeroCross=off  InputSameDT=on
  fc : Outport  VectorParamsAs1DForOutWhenUnconnected=off
  wires:
  FaultCounter/1(count) -> Unit Delay/1
  Unit Delay/1 -> FaultCounter/2(count_prev), Compare To Zero/1
  fc_level/1 -> DTC3/1
  reset/1 -> DTC1/1
  fl/1 -> DTC/1
  FaultCounter/2(fc) -> Signal Conversion/1
  Logical Operator/1 -> FaultCounter/Enable
  Constant/1 -> Unit Delay1/1
  Unit Delay1/1 -> Logical Operator/2
  Compare To Zero/1 -> Logical Operator1/1
  Logical Operator1/1 -> Logical Operator/1
  Signal Conversion/1 -> fc/1
  DTC/1 -> Logical Operator1/2, inc switch/2
  DTC1/1 -> FaultCounter/4(reset)
  DTC3/1 -> FaultCounter/3(fc_level)
  false_count/1 -> inc switch/3
  true_count/1 -> inc switch/1
  inc switch/1 -> FaultCounter/1(fl)

== system common_lib/Diag/Fault Counter w Hold ==
  note: Common Library::Diagnostics::Fault Counter with Hold
  fl : Inport  OutDataTypeStr=boolean
  hold : Inport  Port=2
  true_count : Inport  Port=3
  false_count : Inport  Port=4
  fc_level : Inport  Port=5
  reset : Inport  Port=6  OutDataTypeStr=boolean
  Constant1 : Constant  Value=ZERO
  Constant2 : Constant  Value=false
  Constant3 : Constant  Value=true
  Constant4 : Constant  Value=ZERO
  Constant5 : Constant  Value=false
  Constant6 : Constant  Value=ZERO
  Logical Operator : Logic  Operator=OR
  Relay : $bdroot/Slink/Relay  init=false
      settings: AttributesFormatString=ic=%<init>
  Sat : $bdroot/Slink/Sat
  Sum : Sum  Inputs=++|  InputSameDT=on  OutDataTypeStr=Inherit: Same as first input
  Unit Delay : UnitDelay  InitialCondition=ZERO  SampleTime=-1  HasFrameUpgradeWarning=on
      settings: AttributesFormatString=ic=%<X0>
  Unit Delay1 : UnitDelay  InitialCondition=true  SampleTime=-1  HasFrameUpgradeWarning=on
      settings: AttributesFormatString=ic=%<X0>
  inc switch : Switch  Threshold=0.5  ZeroCross=off  InputSameDT=on
  inc switch1 : Switch  Threshold=0.5  ZeroCross=off  InputSameDT=on
  reset switch1 : Switch  Threshold=0.5  ZeroCross=off  InputSameDT=on
  fc : Outport  VectorParamsAs1DForOutWhenUnconnected=off
  wires:
  inc switch1/1 -> Sum/2
  Constant4/1 -> inc switch1/1
  hold/1 -> inc switch1/2
  Sum/1 -> reset switch1/3
  Constant6/1 -> reset switch1/1
  Relay/1 -> fc/1
  Constant3/1 -> Relay/4
  Constant2/1 -> Relay/5
  Constant1/1 -> Relay/3, Sat/3
  fc_level/1 -> Relay/2, Sat/2
  Sat/1 -> Unit Delay/1
  inc switch/1 -> inc switch1/3
  true_count/1 -> inc switch/1
  fl/1 -> inc switch/2
  false_count/1 -> inc switch/3
  Constant5/1 -> Unit Delay1/1
  Unit Delay1/1 -> Logical Operator/2
  reset/1 -> Logical Operator/1
  Logical Operator/1 -> reset switch1/2
  Unit Delay/1 -> Sum/1
  reset switch1/1 -> Relay/1, Sat/1

== system common_lib/Diag/Fault Injection ==
  note: Common Library::Diagnostics::Fault Injection
  input : Inport
  gain : Inport  Port=2
  offset : Inport  Port=3
  ulim : Inport  Port=4
  llim : Inport  Port=5
  hold : Inport  Port=6
  fl_trigger : Inport  Port=7
  Gain and Offset (in) : $bdroot/SCond/Gain and Offset (in)  DataType=Double
  OOR Fault Detection : $bdroot/Diag/OOR Fault Detection  InitialValue=InitialValue
  Switch : Switch  Threshold=0.5  ZeroCross=off
  Unit Delay : UnitDelay  InitialCondition=InitialValue  SampleTime=-1  HasFrameUpgradeWarning=on
  output : Outport  VectorParamsAs1DForOutWhenUnconnected=off
  hwfl : Outport  Port=2  VectorParamsAs1DForOutWhenUnconnected=off
  wires:
  Gain and Offset (in)/1 -> Switch/3
  Switch/1 -> OOR Fault Detection/1
  Unit Delay/1 -> Switch/1
  hold/1 -> Switch/2
  llim/1 -> OOR Fault Detection/3
  ulim/1 -> OOR Fault Detection/2
  fl_trigger/1 -> OOR Fault Detection/4
  OOR Fault Detection/2 -> hwfl/1
  OOR Fault Detection/1 -> Unit Delay/1, output/1
  offset/1 -> Gain and Offset (in)/3
  gain/1 -> Gain and Offset (in)/2
  input/1 -> Gain and Offset (in)/1

== system common_lib/Diag/Fault Log ==
  note: Common Library::Diagnostics::Fault Log
  HWfl_Active : Inport  OutDataTypeStr=boolean
  HWfl_Events : Inport  Port=2  OutDataTypeStr=uint16
  HWfl_Frames : Inport  Port=3  OutDataTypeStr=uint32
  hold : Inport  Port=4  OutDataTypeStr=boolean
  Constant1 : Constant  Value=EVENT_ZERO
  Constant18 : Constant  Value=EVENT_MAX
  Constant2 : Constant  Value=EVENT_ONE
  Constant3 : Constant  Value=FRAME_ZERO
  Constant4 : Constant  Value=FRAME_MAX
  Constant5 : Constant  Value=FRAME_ONE
  Logical Operator1 : Logic
  Logical Operator3 : Logic
  Logical Operator8 : Logic
  Sat : $bdroot/Slink/Sat
  Sat1 : $bdroot/Slink/Sat
  Sum : Sum  Inputs=|++  InputSameDT=on  OutDataTypeStr=Inherit: Same as first input
  Sum1 : Sum  Inputs=|++  InputSameDT=on  OutDataTypeStr=Inherit: Same as first input
  Unit Delay1 : UnitDelay  InitialCondition=false  SampleTime=-1  HasFrameUpgradeWarning=on
  not1 : Logic  Operator=NOT
  not2 : Logic  Operator=NOT
  reset switch : Switch  Criteria=u2 ~= 0  Threshold=0.5  ZeroCross=off  InputSameDT=on
  reset switch1 : Switch  Criteria=u2 ~= 0  Threshold=0.5  ZeroCross=off  InputSameDT=on
  events : Outport  VectorParamsAs1DForOutWhenUnconnected=off
  frames : Outport  Port=2  VectorParamsAs1DForOutWhenUnconnected=off
  wires:
  Logical Operator3/1 -> reset switch/2
  Logical Operator8/1 -> not1/1, Logical Operator3/1
  Unit Delay1/1 -> Logical Operator3/2
  not1/1 -> Unit Delay1/1
  Logical Operator1/1 -> reset switch1/2
  hold/1 -> not2/1
  not2/1 -> Logical Operator8/2, Logical Operator1/1
  HWfl_Frames/1 -> Sum1/2, reset switch1/3
  HWfl_Events/1 -> Sum/2, reset switch/3
  Constant5/1 -> Sum1/1
  Sat1/1 -> frames/1
  Sum1/1 -> reset switch1/1
  reset switch1/1 -> Sat1/1
  Constant3/1 -> Sat1/3
  Constant4/1 -> Sat1/2
  Constant2/1 -> Sum/1
  Sat/1 -> events/1
  Sum/1 -> reset switch/1
  reset switch/1 -> Sat/1
  Constant1/1 -> Sat/3
  Constant18/1 -> Sat/2
  HWfl_Active/1 -> Logical Operator1/2, Logical Operator8/1

== system common_lib/Diag/Fault_Cntr ==
  note: Common Library::Diagnostics::Fault Counter
  fl : Inport  OutDataTypeStr=boolean
  reset : Inport  Port=2  OutDataTypeStr=boolean
  fmi : Inport  Port=3  OutDataTypeStr=uint16
  Constant1 : Constant  Value=up_cnt
  Constant10 : Constant  Value=red_light  OutDataTypeStr=boolean
  Constant2 : Constant  Value=dn_cnt
  Constant3 : Constant  Value=fc_level  OutDataTypeStr=int16
  Constant4 : Constant  Value=fault_id  OutDataTypeStr=uint16
  Constant6 : Constant  Value=amber_light  OutDataTypeStr=boolean
  Data Type Conversion : DataTypeConversion  OutDataTypeStr=uint16
  Data Type Conversion1 : DataTypeConversion  OutDataTypeStr=boolean
  Data Type Conversion2 : DataTypeConversion  OutDataTypeStr=int16
  Data Type Conversion3 : DataTypeConversion  OutDataTypeStr=int16
  FaultHandlerCoreLogic : Subsystem  TreatAsAtomicUnit=on  RTWFcnName=FC_FMI_Handler
      settings: RTWFcnNameOpts=User specified  RTWFileNameOpts=Use function name
  Signal Conversion : SignalConversion  ConversionOutput=Contiguous copy  OverrideOpt=on
  Signal Conversion1 : SignalConversion  ConversionOutput=Contiguous copy  OverrideOpt=on
  inc switch : Switch  Criteria=u2 ~= 0  Threshold=0.5  ZeroCross=off  InputSameDT=on
  fc : Outport  OutDataTypeStr=uint16  VectorParamsAs1DForOutWhenUnconnected=off
  lights : Outport  Port=2  OutDataTypeStr=uint8  VectorParamsAs1DForOutWhenUnconnected=off
  wires:
  fl/1 -> inc switch/2
  reset/1 -> Data Type Conversion1/1
  FaultHandlerCoreLogic/1(fc) -> Signal Conversion/1
  fmi/1 -> Data Type Conversion/1
  FaultHandlerCoreLogic/2(lights) -> Signal Conversion1/1
  Signal Conversion/1 -> fc/1
  Signal Conversion1/1 -> lights/1
  Data Type Conversion/1 -> FaultHandlerCoreLogic/3(fmi)
  Data Type Conversion1/1 -> FaultHandlerCoreLogic/2(reset)
  Constant2/1 -> inc switch/3
  Constant3/1 -> Data Type Conversion3/1
  Constant4/1 -> FaultHandlerCoreLogic/5(fid)
  Constant10/1 -> FaultHandlerCoreLogic/6(red)
  Constant6/1 -> FaultHandlerCoreLogic/7(amber)
  Constant1/1 -> inc switch/1
  inc switch/1 -> Data Type Conversion2/1
  Data Type Conversion2/1 -> FaultHandlerCoreLogic/1(fl)
  Data Type Conversion3/1 -> FaultHandlerCoreLogic/4(fc_level)

== system common_lib/Diag/Filter w Fault Handler ==
  input : Inport
  tau : Inport  Port=2
  override_value : Inport  Port=3
  override? : Inport  Port=4
  reset? : Inport  Port=5
  default : Inport  Port=6
  ramp_time : Inport  Port=7
  fault? : Inport  Port=8
  Data Type Conversion{,1..4} (5 alike) : DataTypeConversion  OutDataTypeStr=single
  Data Type Conversion5 : DataTypeConversion  OutDataTypeStr=boolean
  Data Type Conversion6 : DataTypeConversion  OutDataTypeStr=boolean
  Data Type Conversion7 : DataTypeConversion  OutDataTypeStr=boolean
  FilterWithFaultHandlerCoreLogic : Subsystem  TreatAsAtomicUnit=on  RTWFcnName=FLTRWROFH
      settings: RTWFcnNameOpts=User specified  RTWFileNameOpts=Use function name
  Signal Conversion : SignalConversion  ConversionOutput=Contiguous copy  OverrideOpt=on
  output : Outport  VectorParamsAs1DForOutWhenUnconnected=off
  wires:
  input/1 -> Data Type Conversion/1
  tau/1 -> Data Type Conversion1/1
  override_value/1 -> Data Type Conversion2/1
  FilterWithFaultHandlerCoreLogic/1(output) -> Signal Conversion/1
  override?/1 -> Data Type Conversion7/1
  reset?/1 -> Data Type Conversion6/1
  default/1 -> Data Type Conversion3/1
  ramp_time/1 -> Data Type Conversion4/1
  fault?/1 -> Data Type Conversion5/1
  Signal Conversion/1 -> output/1
  Data Type Conversion/1 -> FilterWithFaultHandlerCoreLogic/1(input)
  Data Type Conversion1/1 -> FilterWithFaultHandlerCoreLogic/2(tau)
  Data Type Conversion2/1 -> FilterWithFaultHandlerCoreLogic/3(override_value)
  Data Type Conversion3/1 -> FilterWithFaultHandlerCoreLogic/6(default)
  Data Type Conversion4/1 -> FilterWithFaultHandlerCoreLogic/7(ramp_time)
  Data Type Conversion5/1 -> FilterWithFaultHandlerCoreLogic/8(fault?)
  Data Type Conversion6/1 -> FilterWithFaultHandlerCoreLogic/5(reset?)
  Data Type Conversion7/1 -> FilterWithFaultHandlerCoreLogic/4(override?)

== system common_lib/Diag/Filter w Fault Handler1 ==
  note: Common Library::Diagnostics::Filter With Fault Handler
  input : Inport
  tau : Inport  Port=2
  reset? : Inport  Port=3
  default : Inport  Port=4
  ramp_time : Inport  Port=5
  fault? : Inport  Port=6
  Abs1 : Abs  ZeroCross=off
  Abs2 : Abs  ZeroCross=off
  Constant5 : Constant  Value=TimeStep
  Fltr_wRO : Subsystem  RTWFcnName=FLTRWRO  mask(CL Filter wRO){TimeStep=TimeStep}
      mask prompts: TimeStep "Time Step"
      mask help:
      | First Order Filter, y(n)= T/tau x(n) + (1 - T/tau) y(n-1)
      |
      | If override is true (1) then output=override_value
      | If      reset is true (1) then output=input
      |    otherwise output = previous output + (input - previous output) * T/tau
      |
      | X(1) = input
      | X(2) = tau
      | X(3) = override value
      | X(4) = override flag
      | X(5) = reset flag
      |
      | Y(1) = output
      |
      | Time step is entered via mask parameter.
      | NgEK, Inc.
      mask init:
      | switch class(TimeStep)
      |  case ('double')
      |       IC = double(0.0);
      |     case ('single')
      |        IC = single(0.0);
      |     case ('int8')
      |          IC = int8(0);
      |     case ('int16')
      |       IC = int16(0);
      |    case ('int32')
      |         IC = int32(0);
      | end;
      settings: RTWFileNameOpts=Use function name
      mask Help: web(which(['common_lib17.html']))
      mask Display:
      | patch([0.4 0.4 0.6 0.6], [0.35 0.65 0.65 0.35], [255/255 127/255 255/255])
      | disp('Filter\nw RO')
      | port_label('input', 1, 'input')
      | port_label('input', 2, 'tau')
      | port_label('input', 3, 'override_value')
      | port_label('input', 4, 'override?')
      | port_label('input', 5, 'reset?')
      | port_label('output', 1, 'output')
  Product1 : Product  Inputs=**/  InputSameDT=on  OutDataTypeStr=Inherit: Same as first input
  Sum1 : Sum  Inputs=+-|  InputSameDT=on  OutDataTypeStr=Inherit: Same as first input
  Sum2 : Sum  Inputs=+-|  InputSameDT=on  OutDataTypeStr=Inherit: Same as first input
  Sum3 : Sum  Inputs=+-|  InputSameDT=on  OutDataTypeStr=Inherit: Same as first input
  Switch{1..4} (4 alike) : Switch  Threshold=0.5  ZeroCross=off  InputSameDT=on
  delay : UnitDelay  InitialCondition=Zero  SampleTime=-1  HasFrameUpgradeWarning=on
  ic: signal at fault : UnitDelay  InitialCondition=Zero  SampleTime=-1  HasFrameUpgradeWarning=on
  within zero tol of corrections : RelationalOperator  Operator=<  ZeroCross=off  RndMeth=Nearest
  output : Outport  VectorParamsAs1DForOutWhenUnconnected=off
  wires:
  Sum3/1 -> Abs1/1
  delay/1 -> Switch2/1
  Switch3/1 -> delay/1
  within zero tol of corrections/1 -> Switch3/2
  Abs2/1 -> within zero tol of corrections/1
  Abs1/1 -> within zero tol of corrections/2
  Sum2/1 -> Switch3/1
  Switch1/1 -> Sum3/1, Sum2/1
  Switch4/1 -> Switch1/3, Sum1/1, ic: signal at fault/1
  ic: signal at fault/1 -> Switch4/1
  Product1/1 -> Abs2/1, Sum2/2
  Constant5/1 -> Product1/2
  Sum1/1 -> Product1/1
  default/1 -> Sum3/2, Switch3/3, Sum1/2
  Fltr_wRO/1(output) -> Switch4/3, output/1
  input/1 -> Switch2/3
  Switch2/1 -> Switch1/1, Fltr_wRO/1(input)
  reset?/1 -> Fltr_wRO/3(reset?)
  tau/1 -> Fltr_wRO/2(tau)
  fault?/1 -> Switch1/2, Switch4/2, Switch2/2
  ramp_time/1 -> Product1/3

== system common_lib/Diag/OOR Fault Detection ==
  note: Common Library::Diagnostics::Out of Range Fault Detection
  in : Inport
  ulim : Inport  Port=2
  llim : Inport  Port=3
  ext_fault? : Inport  Port=4
  Logical Operator : Logic  Operator=OR  Inputs=3  AllPortsSameDT=off
  Relational Operator : RelationalOperator  Operator=<  ZeroCross=off  RndMeth=Nearest
  Relational Operator1 : RelationalOperator  Operator=<  ZeroCross=off  RndMeth=Nearest
  Sat : $bdroot/Slink/Sat
  Switch : Switch  Threshold=0.5  ZeroCross=off
  Unit Delay : UnitDelay  InitialCondition=InitialValue  SampleTime=-1  HasFrameUpgradeWarning=on
  out : Outport  VectorParamsAs1DForOutWhenUnconnected=off
  fault? : Outport  Port=2  VectorParamsAs1DForOutWhenUnconnected=off
  wires:
  Sat/1 -> Unit Delay/1, out/1
  Switch/1 -> Sat/1
  ext_fault?/1 -> Logical Operator/3
  llim/1 -> Sat/3, Relational Operator/2
  ulim/1 -> Relational Operator1/1, Sat/2
  in/1 -> Relational Operator1/2, Relational Operator/1, Switch/3
  Relational Operator1/1 -> Logical Operator/1
  Relational Operator/1 -> Logical Operator/2
  Logical Operator/1 -> Switch/2, fault?/1
  Unit Delay/1 -> Switch/1

== system common_lib/Diag/Rate Limit Fault Detection ==
  note: Common Library::Diagnostics::Rate Limit Fault Detection
  in : Inport
  rlim : Inport  Port=2
  ext_fault? : Inport  Port=3
  Constant1 : Constant  Value=true
  Constant2 : Constant  Value=TimeStep
  Data Type Conversion : DataTypeConversion  OutDataTypeStr=single
  OOR Fault Detection : $bdroot/Diag/OOR Fault Detection  InitialValue=IC
  Product1 : Product  InputSameDT=on  OutDataTypeStr=Inherit: Same as first input
  Sum1 : Sum  Inputs=-+|  InputSameDT=on  OutDataTypeStr=Inherit: Same as first input
  Sum2 : Sum  Inputs=|++  InputSameDT=on  OutDataTypeStr=Inherit: Same as first input
  Sum3 : Sum  Inputs=++|  InputSameDT=on  OutDataTypeStr=Inherit: Same as first input
  Unit Delay : UnitDelay  InitialCondition=Zero  SampleTime=-1  HasFrameUpgradeWarning=on
      settings: AttributesFormatString=ic=%<X0>
  Unit Delay1 : UnitDelay  InitialCondition=false  SampleTime=-1  HasFrameUpgradeWarning=on
      settings: AttributesFormatString=ic=%<X0>
  Unit Delay2 : UnitDelay  InitialCondition=Zero  SampleTime=-1  HasFrameUpgradeWarning=on
      settings: AttributesFormatString=ic=%<X0>
  Unit Delay3 : UnitDelay  InitialCondition=false  SampleTime=-1  HasFrameUpgradeWarning=on
      settings: AttributesFormatString=ic=%<X0>
  inc switch : Switch  Threshold=0.5  ZeroCross=off  InputSameDT=on
  inc switch1 : Switch  Threshold=0.5  ZeroCross=off  InputSameDT=on
  out : Outport  VectorParamsAs1DForOutWhenUnconnected=off
  fault? : Outport  Port=2  VectorParamsAs1DForOutWhenUnconnected=off
  wires:
  Constant2/1 -> Data Type Conversion/1
  Data Type Conversion/1 -> Product1/1
  inc switch1/1 -> Sum2/1, Sum1/2
  Unit Delay3/1 -> inc switch1/2
  Constant1/1 -> Unit Delay3/1
  Unit Delay/1 -> inc switch1/1
  Unit Delay1/1 -> inc switch/2
  Unit Delay2/1 -> Sum3/1
  Sum3/1 -> inc switch/1
  Product1/1 -> Sum3/2, inc switch/3
  rlim/1 -> Product1/2
  inc switch/1 -> Unit Delay2/1, Sum1/1, Sum2/2
  Sum2/1 -> OOR Fault Detection/2
  Sum1/1 -> OOR Fault Detection/3
  OOR Fault Detection/2 -> Unit Delay1/1, fault?/1
  OOR Fault Detection/1 -> Unit Delay/1, out/1
  ext_fault?/1 -> OOR Fault Detection/4
  in/1 -> inc switch1/3, OOR Fault Detection/1
